simulink model "pendule_inv_etu"  (R2022a)
settings: Solver=VariableStepAuto  StartTime=0.0  StopTime=10.0  RelTol=1e-3
values from neighbouring files (symbols this model uses):
  g = 9.81    [simu_pendule_inv_capteur_etu.m]    (also in simu_pendule_inv_echant_etu.m; simu_pendule_inv_etu.m)
  K = [10 1]    [simu_pendule_inv_capteur_etu.m]    (also in simu_pendule_inv_echant_etu.m = [30 10]; simu_pendule_inv_etu.m = [30 10])
  l = 10    [simu_pendule_inv_capteur_etu.m]    (also in simu_pendule_inv_echant_etu.m; simu_pendule_inv_etu.m)
  ue = 0    [simu_pendule_inv_capteur_etu.m]    (also in simu_pendule_inv_echant_etu.m; simu_pendule_inv_etu.m)
  x0 = [pi/20 0]'    [simu_pendule_inv_capteur_etu.m]    (also in simu_pendule_inv_echant_etu.m; simu_pendule_inv_etu.m = [pi/10 0]')
  xe = [0 0]'    [simu_pendule_inv_capteur_etu.m]    (also in simu_pendule_inv_echant_etu.m; simu_pendule_inv_etu.m)
settings Model: Creator=paul  LastModifiedBy=paul
settings ModelReferenceCC: EnableRefExpFcnMdlSchedulingChecks=off
settings RTWCC: Description=Generic Real-Time Target

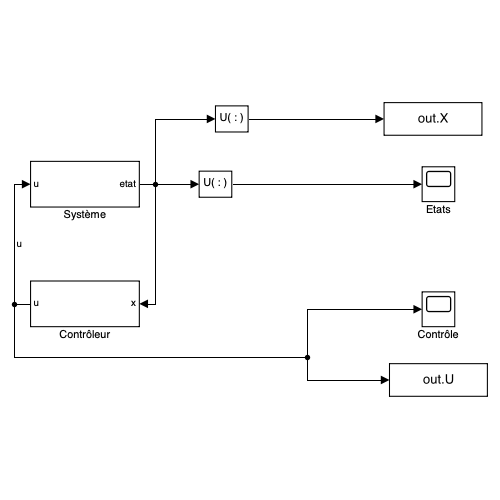
[thumbnail: Simulink's stored preview of the top-level diagram]
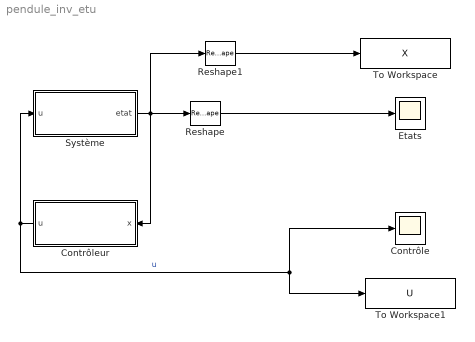
== system pendule_inv_etu ==
  Contrôle : Scope
  Contrôleur : Subsystem
  Etats : Scope
  Reshape : Reshape
  Reshape1 : Reshape
  Système : Subsystem
  To Workspace : ToWorkspace  VariableName=X  SaveFormat=Timeseries  SampleTime=-1
  To Workspace1 : ToWorkspace  VariableName=U  SaveFormat=Timeseries  SampleTime=-1
  wires:
  Système/1(etat) -> Contrôleur/1(x), Reshape/1, Reshape1/1
  Contrôleur/1(u) -> Contrôle/1, To Workspace1/1, Système/1(u)  "u"
  Reshape/1 -> Etats/1
  Reshape1/1 -> To Workspace/1

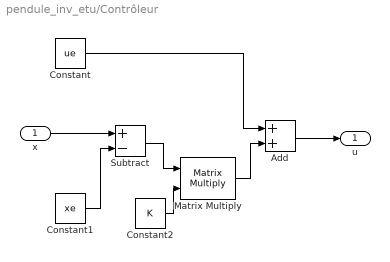
== system pendule_inv_etu/Contrôleur ==
  x : Inport
  Add : Sum
  Constant : Constant  Value=ue
  Constant1 : Constant  Value=xe
  Constant2 : Constant  Value=K
  Matrix Multiply : Product  Multiplication=Matrix(*)
  Subtract : Sum  Inputs=+-
  u : Outport
  wires:
  x/1 -> Subtract/1
  Constant1/1 -> Subtract/2
  Subtract/1 -> Matrix Multiply/1
  Constant/1 -> Add/1
  Matrix Multiply/1 -> Add/2
  Add/1 -> u/1
  Constant2/1 -> Matrix Multiply/2

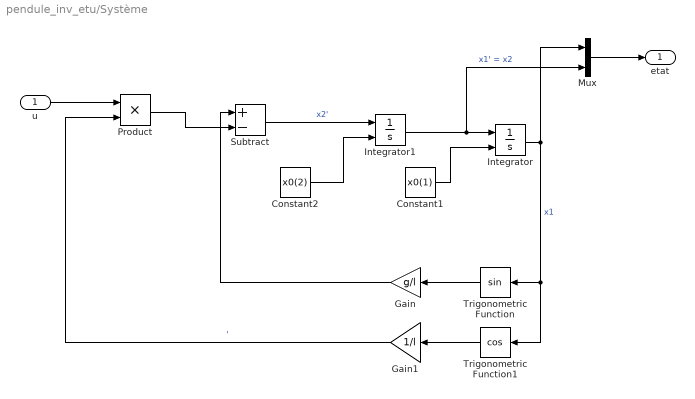
== system pendule_inv_etu/Système ==
  u : Inport
  Constant1 : Constant  Value=x0(1)
  Constant2 : Constant  Value=x0(2)
  Gain : Gain  Gain=g/l
  Gain1 : Gain  Gain=1/l
  Integrator : Integrator  InitialConditionSource=external
  Integrator1 : Integrator  InitialConditionSource=external
  Mux : Mux  Inputs=2
  Product : Product
  Subtract : Sum  Inputs=+-
  Trigonometric Function : Trigonometry
  Trigonometric Function1 : Trigonometry  Operator=cos
  etat : Outport
  wires:
  Integrator/1 -> Mux/1, Trigonometric Function/1, Trigonometric Function1/1  "x1"
  Integrator1/1 -> Mux/2, Integrator/1  "x1' = x2"
  Trigonometric Function/1 -> Gain/1
  Trigonometric Function1/1 -> Gain1/1
  u/1 -> Product/1
  Subtract/1 -> Integrator1/1  "x2'"
  Gain1/1 -> Product/2  "'"
  Constant1/1 -> Integrator/2
  Constant2/1 -> Integrator1/2
  Mux/1 -> etat/1
  Gain/1 -> Subtract/1
  Product/1 -> Subtract/2
